simulink model "Simulaciones_punto_5"  (R2017a)
settings: Solver=VariableStepAuto  StartTime=0.0  StopTime=5  RelTol=1e-3
settings Model: Creator=franj  LastModifiedBy=franj

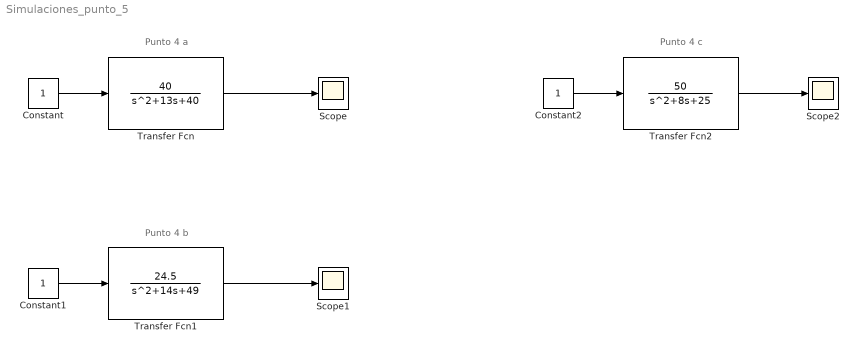
== system Simulaciones_punto_5 ==
  note: Punto 4 b
  note: Punto 4 a
  note: Punto 4 c
  Constant : Constant
  Constant1 : Constant
  Constant2 : Constant
  Scope : Scope
  Scope1 : Scope
  Scope2 : Scope
  Transfer Fcn : TransferFcn  Numerator=[40]  Denominator=[1 13 40]
  Transfer Fcn1 : TransferFcn  Numerator=[24.5]  Denominator=[1 14 49]
  Transfer Fcn2 : TransferFcn  Numerator=[50]  Denominator=[1 8 25]
  wires:
  Constant/1 -> Transfer Fcn/1
  Transfer Fcn/1 -> Scope/1
  Transfer Fcn1/1 -> Scope1/1
  Constant1/1 -> Transfer Fcn1/1
  Transfer Fcn2/1 -> Scope2/1
  Constant2/1 -> Transfer Fcn2/1
